simulink model "parc_simu"  (R2015a)
settings: Solver=ode45  StartTime=0.0  StopTime=100  RelTol=1e-3
values from neighbouring files (symbols this model uses):
  Kpexp = -0.6    [codigo_3_ROLDAN.m]
libraries: cstblocks x1
settings Model: Creator=Jose Roldan  LastModifiedBy=Jose Roldan

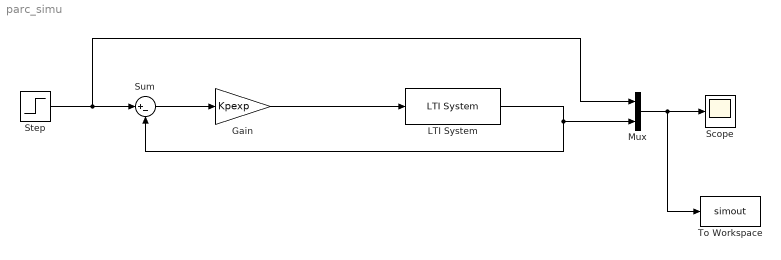
== system parc_simu ==
  Gain : Gain  Gain=Kpexp
  LTI System : cstblocks/LTI System  sys=G  IC=[]
  Mux : Mux  Inputs=2
  Scope : Scope
  Step : Step  SampleTime=0
  Sum : Sum  Inputs=|+-
  To Workspace : ToWorkspace  VariableName=simout  SaveFormat=Timeseries  SampleTime=-1
  wires:
  Gain/1 -> LTI System/1
  LTI System/1 -> Mux/2, Sum/2
  Step/1 -> Mux/1, Sum/1
  Sum/1 -> Gain/1
  Mux/1 -> To Workspace/1, Scope/1
